simulink model "RL_TTS3_Controller_Blank"  (R2019b)
settings: Solver=FixedStepAuto  StartTime=0.0  StopTime=10.0  FixedStep=0.01  RelTol=1e-3
PostLoadFcn:
  | if any(exist('dsrtsu_mdlpostloadfcn', 'file') ~= 0), dsrtsu_mdlpostloadfcn('Execute', bdroot); end
values from neighbouring files (symbols this model uses):
  Dvalve = sqrt(4*S/pi)    [determining.m]    (also in nonTunables.mat = 0.00797884560803)
  K = [12.980610275 0.418319912 -2.0948707556 3.01551653144 0.41832512629 13.0045004905 2.89259412877 -2.22453205977 3.90699303281 3.7610923526 21.5549448701 21.6369062336 ... (20 elements, 4x5)]    [nonTunables.mat]
  Ts = 0.01    [RL_TTS3_Controller_Blank.mat]    (also in determining.m = 0.01;67)
libraries: simulink x5
settings Model: DSRTSU_INTERNAL_RTI_VER=550  DSRTSU_INTERNAL_RTI_TYPE=rti1104  RTICANMMDATA=struct('GeneralSetupData',struct('modelroot','E:\Will\RemoteLabs\TTS3\HostPC','generalsettings',struct('filesettings',struct('destfolder',struct('Name','RTICANMM_FILES','Check',1),'buildfolder',struct('Name','.','Check',1),'AbsDestfolder',struct('Name','E:\Will\RemoteLabs\TTS3\HostPC\RTICANMM_FILES'),'AbsBuildfolder',struct('Name','E:\Will\RemoteLabs\TTS3\HostPC'))),'options',struct('addpaths',1,'rmpaths',1,'addtrcexclusion',true,'cannavigator',struct('checkmonitoring',0),'show_usrtrc',0,'use_usrtrc',0),'advanced',struct('options',ones(1,100)),'MPSetup',{{}},'RTI',struct('Type','RTI1104','Ver','7.13','Date','02-Nov-2019'),'modelname','TTS3_Controller_Test_OL','block','TTS3_Controller_Test_OL'))  DSRTSU_INTERNAL_RTIFPGA=150  Creator=whendrix  LastModifiedBy=maxva
settings OptimizationCC: BlockReduction=off  DefaultParameterBehavior=Inlined  OptimizeBlockIOStorage=off  BufferReuse=off  GlobalBufferReuse=off  ExpressionFolding=off  LocalBlockOutputs=off  OptimizeDataStoreBuffers=off  BusAssignmentInplaceUpdate=off
settings DebuggingCC: BusObjectLabelMismatch=none
settings HardwareCC: ProdBitPerPointer=32  ProdBitPerSizeT=32  ProdBitPerPtrDiffT=32  ProdLargestAtomicInteger=Integer  ProdEndianess=BigEndian  ProdWordSize=32  ProdHWDeviceType=Custom Processor->Custom  TargetIntDivRoundTo=Zero  TargetEndianess=BigEndian  TargetHWDeviceType=Custom Processor->Custom
settings ModelReferenceCC: ModelReferenceNumInstancesAllowed=Single  ModelReferenceMinAlgLoopOccurrences=on
settings SFSimCC: MATLABDynamicMemAlloc=off  CustomCodeUndefinedFunction=UseInterfaceOnly
settings RTWCC: Description=dSPACE DS1104 Hardware Platform  SystemTargetFile=rti1104.tlc  MakeCommand=make_rti  TemplateMakefile=rti1104.tmf
settings CodeAppCC: MaxIdLength=63
settings STFCustomTargetCC: ParMdlRefBuildCompliant=on  SystemTargetFile=rti1104.tlc
settings GRTTargetCC: TargetLangStandard=C89/C90 (ANSI)  CompOptLevelCompliant=off  ConcurrentExecutionCompliant=off  CombineOutputUpdateFcns=off  MatFileLogging=off  CPPClassGenCompliant=off  UseToolchainInfoCompliant=off

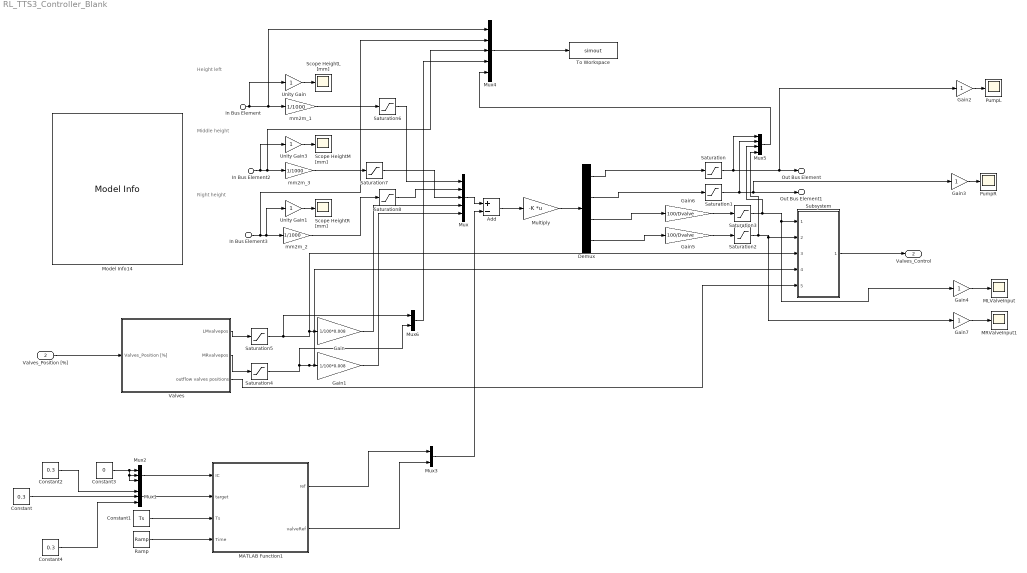
== system RL_TTS3_Controller_Blank ==
  note: Height left
  note: Middle height
  note: Right height
  In Bus Element : Inport  PortName=Heights [mm]  Element=Left
  In Bus Element2 : Inport  PortName=Heights [mm]  Element=Middle
  In Bus Element3 : Inport  PortName=Heights [mm]  Element=Right
  Valves_Position [%] : Inport  Port=2  OutDataTypeStr=Bus: ValvesSOCI
  Add : Sum  Inputs=+-
  Constant : Constant  Value=0.3
  Constant1 : Constant  Value=Ts
  Constant2 : Constant  Value=0.3
  Constant3 : Constant  Value=0
  Constant4 : Constant  Value=0.3
  Demux : Demux
  Gain : Gain  Gain=1/100*0.008
  Gain1 : Gain  Gain=1/100*0.008
  Gain{2..4,7} (4 alike) : Gain
  Gain5 : Gain  Gain=100/Dvalve
  Gain6 : Gain  Gain=100/Dvalve
  MATLAB Function1 : MATLAB Function  TreatAsAtomicUnit=on
  MLValveInput : Scope
  MRValveInput1 : Scope
  Model Info14 : simulink/Model-Wide Utilities/Model Info  Frame=on  DisplayStringWithTags=|  HorizontalTextAlignment=Left  LeftAlignmentValue=0.02
      | Start model for the "Three Tank"
      | experiment on the "Three Tank" setup.
      | Version: 1.0
      | 
      | 
      | INFORMATION
      | ----------------------
      | 
      | Unity Gain block before Scope is needed for
      | RemoteLabs compatebility. 
      | Do not modify or remove!
      | 
      | Pump range:
      | 0 to 0.102 [l/s]
      | 
      | The 5 Valves are labeled according 
      | to their position:
      | 
      |    LM  MR
      |      X     X
      |  X      X      X
      | LD    MD   RD
      | 
      | L = Left
      | M = Middle
      | R = Right
      | D = Down
  Multiply : Gain  Gain=-K  Multiplication=Matrix(K*u)
  Mux : Mux  Inputs=5
  Mux1 : Mux  Inputs=3
  Mux2 : Mux  Inputs=3
  Mux3 : Mux  Inputs=2
  Mux4 : Mux  Inputs=5
  Mux5 : Mux
  Mux6 : Mux  Inputs=2
  PumpL : Scope
  "PumpR " : Scope
  Ramp : simulink/Sources/Ramp  slope=1  start=0  InitialOutput=0
  Saturation : Saturate  UpperLimit=0.1  LowerLimit=0
  Saturation1 : Saturate  UpperLimit=0.1  LowerLimit=0
  Saturation{2..5} (4 alike) : Saturate  UpperLimit=100  LowerLimit=0
  Saturation6 : Saturate  UpperLimit=0.65  LowerLimit=0
  Saturation7 : Saturate  UpperLimit=0.65  LowerLimit=0
  Saturation8 : Saturate  UpperLimit=0.65  LowerLimit=0
  Scope HeightL [mm] : Scope
  Scope HeightM [mm] : Scope
  Scope HeightR [mm] : Scope
  Subsystem : Subsystem
  To Workspace : ToWorkspace  VariableName=simout  SaveFormat=Timeseries  SampleTime=-1
  Unity Gain : Gain
  Unity Gain1 : Gain
  Unity Gain3 : Gain
  Valves : Subsystem  TreatAsAtomicUnit=on
  mm2m_1 : Gain  Gain=1/1000
  mm2m_2 : Gain  Gain=1/1000
  mm2m_3 : Gain  Gain=1/1000
  Out Bus Element : Outport  VectorParamsAs1DForOutWhenUnconnected=off  PortName=Pumps [l/s]  Element=Left
  Out Bus Element1 : Outport  VectorParamsAs1DForOutWhenUnconnected=off  PortName=Pumps [l/s]  Element=Right
  Valves_Control : Outport  Port=2  OutDataTypeStr=Bus: ValvesSICO  VectorParamsAs1DForOutWhenUnconnected=off
  wires:
  Unity Gain3/1 -> Scope HeightM [mm]/1
  Unity Gain1/1 -> Scope HeightR [mm]/1
  In Bus Element/1 -> Mux4/1, mm2m_1/1, Unity Gain/1
  In Bus Element2/1 -> Mux4/3, mm2m_3/1, Unity Gain3/1
  In Bus Element3/1 -> Mux4/2, mm2m_2/1, Unity Gain1/1
  Valves_Position [%]/1 -> Valves/1(Valves_Position [%])
  Unity Gain/1 -> Scope HeightL [mm]/1
  Subsystem/1(Valves1) -> Valves_Control/1
  Valves/1(LMvalvepos) -> Saturation5/1
  Valves/2("MRvalvepos ") -> Saturation4/1
  Gain3/1 -> "PumpR "/1
  Saturation1/1 -> Mux5/2, Gain3/1, Out Bus Element1/1
  Saturation2/1 -> Mux5/4, Gain7/1, Subsystem/2(MRvalveOpen)
  Saturation3/1 -> Mux5/3, Gain4/1, Subsystem/1("MLValveOpen ")
  Saturation/1 -> Mux5/1, Gain2/1, Out Bus Element/1
  Gain2/1 -> PumpL/1
  Demux/3 -> Gain6/1
  Demux/4 -> Gain5/1
  Demux/1 -> Saturation/1
  Demux/2 -> Saturation1/1
  Multiply/1 -> Demux/1
  mm2m_1/1 -> Saturation6/1
  mm2m_3/1 -> Saturation7/1
  mm2m_2/1 -> Saturation8/1
  Gain/1 -> Mux/4
  Gain1/1 -> Mux/5
  Add/1 -> Multiply/1
  Mux/1 -> Add/1
  Gain6/1 -> Saturation3/1
  Saturation4/1 -> Mux6/2, Subsystem/4(MRValvepos), Gain1/1
  Saturation5/1 -> Mux6/1, Subsystem/3(MLValvepos), Gain/1
  Saturation6/1 -> Mux/1
  Gain5/1 -> Saturation2/1
  Constant3/1 -> Mux2/3, Mux2/2, Mux2/1
  Constant2/1 -> Mux1/1
  Constant1/1 -> MATLAB Function1/3(Ts)
  Mux2/1 -> MATLAB Function1/1(IC)
  MATLAB Function1/2(valveRef) -> Mux3/2
  MATLAB Function1/1(ref) -> Mux3/1
  Mux1/1 -> MATLAB Function1/2(target)
  Ramp/1 -> MATLAB Function1/4(Time)
  Saturation7/1 -> Mux/3
  Saturation8/1 -> Mux/2
  Mux3/1 -> Add/2
  Mux4/1 -> To Workspace/1
  Constant/1 -> Mux1/2
  Constant4/1 -> Mux1/3
  Gain4/1 -> MLValveInput/1
  Gain7/1 -> MRValveInput1/1
  Mux5/1 -> Mux4/5
  Mux6/1 -> Mux4/4
  Valves/3(outflow valves positions) -> Subsystem/5(outflow valves positions)

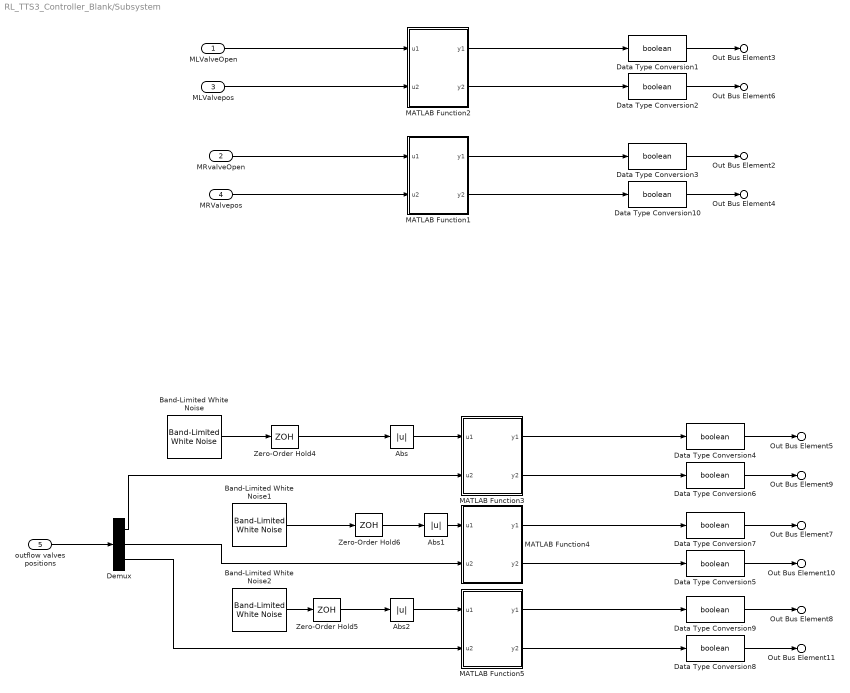
== system RL_TTS3_Controller_Blank/Subsystem ==
  "MLValveOpen " : Inport
  MRvalveOpen : Inport  Port=2
  MLValvepos : Inport  Port=3
  MRValvepos : Inport  Port=4
  outflow valves positions : Inport  Port=5
  Abs : Abs
  Abs1 : Abs
  Abs2 : Abs
  Band-Limited White Noise : simulink/Sources/Band-Limited White Noise  Cov=1000  Ts=10  seed=[23341]
  Band-Limited White Noise1 : simulink/Sources/Band-Limited White Noise  Cov=1000  Ts=10  seed=12345
  Band-Limited White Noise2 : simulink/Sources/Band-Limited White Noise  Cov=1000  Ts=10  seed=[66774]
  Data Type Conversion{1..10} (10 alike) : DataTypeConversion  OutDataTypeStr=boolean
  Demux : Demux  Outputs=3
  MATLAB Function1 : MATLAB Function  TreatAsAtomicUnit=on
  MATLAB Function2 : MATLAB Function  TreatAsAtomicUnit=on
  MATLAB Function3 : MATLAB Function  TreatAsAtomicUnit=on
  MATLAB Function4 : MATLAB Function  TreatAsAtomicUnit=on
  MATLAB Function5 : MATLAB Function  TreatAsAtomicUnit=on
  Zero-Order Hold4 : ZeroOrderHold  SampleTime=Ts
  Zero-Order Hold5 : ZeroOrderHold  SampleTime=Ts
  Zero-Order Hold6 : ZeroOrderHold  SampleTime=Ts
  Out Bus Element8 : Outport  VectorParamsAs1DForOutWhenUnconnected=off  PortName=Valves1  Element=RightDown.Open
  Out Bus Element11 : Outport  VectorParamsAs1DForOutWhenUnconnected=off  PortName=Valves1  Element=RightDown.Close
  Out Bus Element5 : Outport  VectorParamsAs1DForOutWhenUnconnected=off  PortName=Valves1  Element=LeftDown.Open
  Out Bus Element9 : Outport  VectorParamsAs1DForOutWhenUnconnected=off  PortName=Valves1  Element=LeftDown.Close
  Out Bus Element7 : Outport  VectorParamsAs1DForOutWhenUnconnected=off  PortName=Valves1  Element=MiddleDown.Open
  Out Bus Element10 : Outport  VectorParamsAs1DForOutWhenUnconnected=off  PortName=Valves1  Element=MiddleDown.Close
  Out Bus Element2 : Outport  VectorParamsAs1DForOutWhenUnconnected=off  PortName=Valves1  Element=MiddleRight.Open
  Out Bus Element4 : Outport  VectorParamsAs1DForOutWhenUnconnected=off  PortName=Valves1  Element=MiddleRight.Close
  Out Bus Element3 : Outport  VectorParamsAs1DForOutWhenUnconnected=off  PortName=Valves1  Element=LeftMiddle.Open
  Out Bus Element6 : Outport  VectorParamsAs1DForOutWhenUnconnected=off  PortName=Valves1  Element=LeftMiddle.Close
  wires:
  Data Type Conversion4/1 -> Out Bus Element5/1
  Data Type Conversion6/1 -> Out Bus Element9/1
  Data Type Conversion9/1 -> Out Bus Element8/1
  Data Type Conversion8/1 -> Out Bus Element11/1
  Data Type Conversion5/1 -> Out Bus Element10/1
  Data Type Conversion7/1 -> Out Bus Element7/1
  MRvalveOpen/1 -> MATLAB Function1/1(u1)
  MRValvepos/1 -> MATLAB Function1/2(u2)
  "MLValveOpen "/1 -> MATLAB Function2/1(u1)
  MLValvepos/1 -> MATLAB Function2/2(u2)
  Data Type Conversion2/1 -> Out Bus Element6/1
  Data Type Conversion3/1 -> Out Bus Element2/1
  Data Type Conversion10/1 -> Out Bus Element4/1
  Data Type Conversion1/1 -> Out Bus Element3/1
  MATLAB Function4/2(y2) -> Data Type Conversion5/1
  MATLAB Function3/1(y1) -> Data Type Conversion4/1
  MATLAB Function3/2(y2) -> Data Type Conversion6/1
  Demux/2 -> MATLAB Function4/2(u2)
  MATLAB Function4/1(y1) -> Data Type Conversion7/1
  Demux/1 -> MATLAB Function3/2(u2)
  Band-Limited White Noise/1 -> Zero-Order Hold4/1
  MATLAB Function5/2(y2) -> Data Type Conversion8/1
  MATLAB Function5/1(y1) -> Data Type Conversion9/1
  outflow valves positions/1 -> Demux/1
  Abs/1 -> MATLAB Function3/1(u1)
  Abs1/1 -> MATLAB Function4/1(u1)
  Band-Limited White Noise1/1 -> Zero-Order Hold6/1
  Abs2/1 -> MATLAB Function5/1(u1)
  Band-Limited White Noise2/1 -> Zero-Order Hold5/1
  Demux/3 -> MATLAB Function5/2(u2)
  Zero-Order Hold4/1 -> Abs/1
  Zero-Order Hold5/1 -> Abs2/1
  Zero-Order Hold6/1 -> Abs1/1
  MATLAB Function2/1(y1) -> Data Type Conversion1/1
  MATLAB Function2/2(y2) -> Data Type Conversion2/1
  MATLAB Function1/1(y1) -> Data Type Conversion3/1
  MATLAB Function1/2(y2) -> Data Type Conversion10/1

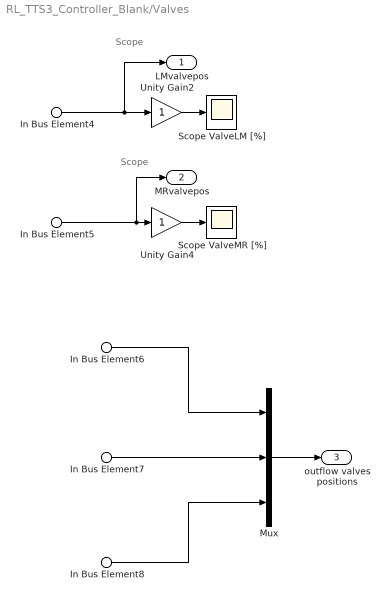
== system RL_TTS3_Controller_Blank/Valves ==
  note: Scope
  note: Scope
  In Bus Element4 : Inport  PortName=Valves_Position [%]  Element=LeftMiddle
  In Bus Element5 : Inport  PortName=Valves_Position [%]  Element=MiddleRight
  In Bus Element6 : Inport  PortName=Valves_Position [%]  Element=LeftDown
  In Bus Element7 : Inport  PortName=Valves_Position [%]  Element=MiddleDown
  In Bus Element8 : Inport  PortName=Valves_Position [%]  Element=RightDown
  Mux : Mux  Inputs=3
  Scope ValveLM [%] : Scope
  Scope ValveMR [%] : Scope
  Unity Gain2 : Gain
  Unity Gain4 : Gain
  LMvalvepos : Outport
  "MRvalvepos " : Outport  Port=2
  outflow valves positions : Outport  Port=3
  wires:
  In Bus Element5/1 -> "MRvalvepos "/1, Unity Gain4/1
  In Bus Element4/1 -> Unity Gain2/1, LMvalvepos/1
  In Bus Element7/1 -> Mux/2
  In Bus Element6/1 -> Mux/1
  In Bus Element8/1 -> Mux/3
  Unity Gain4/1 -> Scope ValveMR [%]/1
  Unity Gain2/1 -> Scope ValveLM [%]/1
  Mux/1 -> outflow valves positions/1

== matlab function RL_TTS3_Controller_Blank/Subsystem/MATLAB Function2 ==
  data: u1 input; y1 output; y2 output; u2 input
function [y1,y2] = fcn(u1,u2)
val = 0.25;
    if abs(u1-u2)<=val % difference is small, set both to false
        y1=false;
        y2 = false;
    elseif u2>u1+val % position is higher than desired position, set close to true and open to false
        y1 = false;
        y2 = true;
    elseif u1>u2+val % desired position is higher than position, set open to true and close to false
        y1 = true;
        y2 = false;
    else
        y1 = false;
        y2 = false;
    end
end

== matlab function RL_TTS3_Controller_Blank/Subsystem/MATLAB Function3 ==
  data: u1 input; y1 output; y2 output; u2 input
function [y1,y2] = fcn(u1,u2)
val = 0.25;
    if abs(u1-u2)<=val
        y1=false;
        y2 = false;
    elseif u2>u1+val
        y1 = false;
        y2 = true;
    elseif u1>u2+val
        y1 = true;
        y2 = false;
    else
        y1 = false;
        y2 = false;
    end
end

== matlab function RL_TTS3_Controller_Blank/Subsystem/MATLAB Function1 ==
  data: u1 input; y1 output; y2 output; u2 input
function [y1,y2] = fcn(u1,u2)
val = 0.25;
    if abs(u1-u2)<=val
        y1=false;
        y2 = false;
    elseif u2>u1+val
        y1 = false;
        y2 = true;
    elseif u1>u2+val
        y1 = true;
        y2 = false;
    else
        y1 = false;
        y2 = false;
    end
end

== matlab function RL_TTS3_Controller_Blank/MATLAB Function1 ==
  data: IC input; ref output; target input; valveRef output; Ts input; Time input
function [ref, valveRef] = fcn(IC, target,Ts,Time)
% input: IC, 3D vector of initial conditions of system
% input: target, 3D vector of target reference for fluid  heights
% input: Sampling time Ts

% output: ref, 3*1 vector containing fluid height references 
% output: valveRef, 2*1 vector containg valve references. Needed for MPC,
% can be ignored (use terminator block in simulink)

%% constants
Atank = 0.0154;
uMaxL = 0.1;        % from Bart's work
uMaxR =  0.09;      % from Bart's work
%% reshaping (check gode generation?)
IC = reshape(IC, [],1);             %  force IC to be a vector
target = reshape(target, [],1);     %  idem
%% calculations
tf = 1.1*sum(target)*Atank/(uMaxL+uMaxR-3*0.01)*1000;  % give a 10% margin for pump dynamics etc, choose 50% of maximum disturbance allowed as 'constant disturbance'
ref = zeros(3,1);
valveRef = zeros(2,1);
matr = [1 zeros(1,3);
        0 1  0    0;
        1 tf tf^2 tf^3;
        0 1 2*tf 3*tf^2];
invmatr = inv(matr);
if  Time < tf
    for i =1:3
        vec = [IC(i);0;target(i);0];
        polyCoeff = invmatr*vec;
        ref(i,1) = polyCoeff(1)+polyCoeff(2)*Time+polyCoeff(3)*Time.^2+polyCoeff(4)*Time.^3;
    end
else
    ref = target;
end

== matlab function RL_TTS3_Controller_Blank/Subsystem/MATLAB Function4 ==
  data: u1 input; y1 output; y2 output; u2 input
function [y1,y2] = fcn(u1,u2)
    if abs(u1-u2)<=2
        y1=false;
        y2 = false;
    elseif u2>u1+2
        y1 = false;
        y2 = true;
    elseif u1>u2+2
        y1 = true;
        y2 = false;
    else
        y1 = false;
        y2 = false;
    end
end

== matlab function RL_TTS3_Controller_Blank/Subsystem/MATLAB Function5 ==
  data: u1 input; y1 output; y2 output; u2 input
function [y1,y2] = fcn(u1,u2)
    if abs(u1-u2)<=2
        y1=false;
        y2 = false;
    elseif u2>u1+2
        y1 = false;
        y2 = true;
    elseif u1>u2+2
        y1 = true;
        y2 = false;
    else
        y1 = false;
        y2 = false;
    end
end
